simulink model "PLL_vs_Hilbert_Mdpi"  (R2024b)
settings: Solver=ode4  StartTime=0.0  StopTime=t(end)  FixedStep=dt  MaxStep=1/10  MinStep=1/10/100  RelTol=1e-3
values from neighbouring files (symbols this model uses):
  case_input = 4    [PLL_script_MDPI.m]
  dt = 1/Fs    (= 0.2)    [Excitation_Force_RM3.m]    (also in PLL_script_MDPI.m = t(2)-t(1); RM3_instf_init.m = round(t(2)-t(1),1); eta2Fex.m = 1/opt.Fs)
  H_s = 2    [PLL_script_MDPI.m]    (also in RM3_instf_init.m)
  median_window = round(2*delay_factor*window_size)    [PLL_script_MDPI.m]    (also in RM3_instf_init.m)
  median_window_seconds = round(0.05*window_size*dt)    [PLL_script_MDPI.m]
  wbar = 2*pi*fp    (= 0.698131700798)    [PLL_script_MDPI.m]    (also in RM3_instf_init.m)
  window_size = round(10*2*pi/wbar/dt)    [PLL_script_MDPI.m]    (also in RM3_instf_init.m)
undefined symbols (not defined in the file or in its folder): A_VCO, window_size_seconds
libraries: simulink x5, dspsigops x4, slpidlib x3, dspxfrm3 x3, dspfdesign x1, dspstat3 x1, eeSinusoidalMeasurementV2 x1
settings Model: Creator=inyongkim  LastModifiedBy=inyongkim
settings OptimizationCC: BlockReduction=off  DefaultParameterBehavior=Inlined  BufferReuse=off

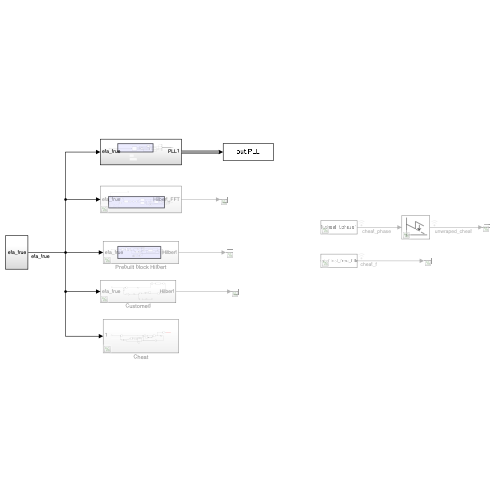
[thumbnail: Simulink's stored preview of the top-level diagram]
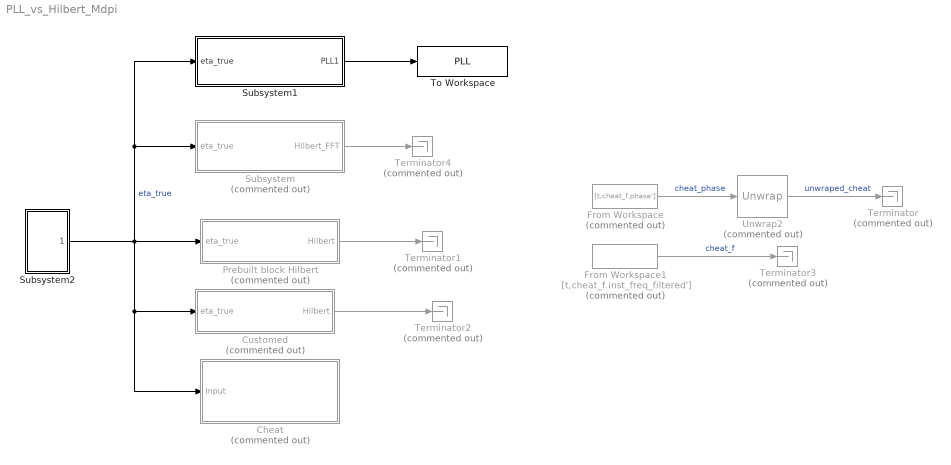
== system PLL_vs_Hilbert_Mdpi ==
  Cheat : Subsystem  Commented=on
  Customed : Subsystem  Commented=on
  From Workspace : FromWorkspace  Commented=on  VariableName=[t,cheat_f.phase']
  From Workspace1 : FromWorkspace  Commented=on  VariableName=[t,cheat_f.inst_freq_filtered']
  Prebuilt block Hilbert : Subsystem  Commented=on
  Subsystem : Subsystem  Commented=on
  Subsystem1 : Subsystem
  Subsystem2 : Subsystem
  Terminator{,1..4} (5 alike) : Terminator  Commented=on
  To Workspace : ToWorkspace  VariableName=PLL  SaveFormat=Timeseries  SampleTime=-1
  Unwrap2 : dspsigops/Unwrap  Commented=on  tol=pi  InputProcessing=Columns as channels (frame based)  running=off
  wires:
  Subsystem/1(Hilbert_FFT) -> Terminator4/1
  Prebuilt block Hilbert/1(Hilbert) -> Terminator1/1
  Subsystem1/1(PLL1) -> To Workspace/1
  Customed/1(Hilbert) -> Terminator2/1
  Subsystem2/1(eta_true) -> Cheat/1(Input), Customed/1(eta_true), Subsystem1/1(eta_true), Subsystem/1(eta_true), Prebuilt block Hilbert/1(eta_true)  "eta_true"
  From Workspace/1 -> Unwrap2/1  "cheat_phase"
  Unwrap2/1 -> Terminator/1  "unwraped_cheat"
  From Workspace1/1 -> Terminator3/1  "cheat_f"

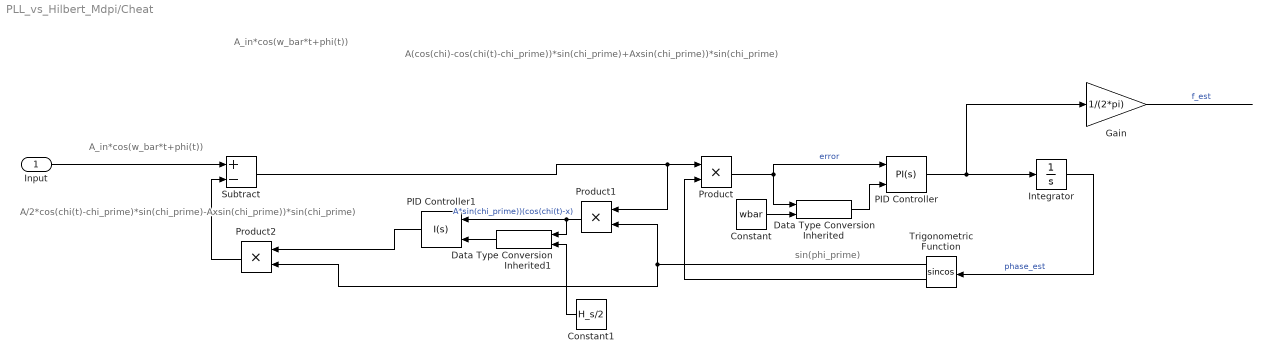
== system PLL_vs_Hilbert_Mdpi/Cheat ==
  note: A/2*cos(chi(t)-chi_prime)*sin(chi_prime)-Axsin(chi_prime))*sin(chi_prime)
  note: sin(phi_prime)
  note: A_in*cos(w_bar*t+phi(t))
  note: A_in*cos(w_bar*t+phi(t))
  note: A(cos(chi)-cos(chi(t)-chi_prime))*sin(chi_prime)+Axsin(chi_prime))*sin(chi_prime)
  Input : Inport
  Constant : Constant  Value=wbar
  Constant1 : Constant  Value=H_s/2
  Data Type Conversion Inherited : simulink/Signal Attributes/Data Type Conversion Inherited  ConvertRealWorld=Real World Value  DoSatur=off
  Data Type Conversion Inherited1 : simulink/Signal Attributes/Data Type Conversion Inherited  ConvertRealWorld=Real World Value  DoSatur=off
  Gain : Gain  Gain=1/(2*pi)
  Integrator : Integrator  LimitOutput=on  UpperSaturationLimit=2*pi  LowerSaturationLimit=0
  PID Controller : slpidlib/PID Controller  Controller=PI  Form=Parallel  TimeDomain=Continuous-time  UseExternalTs=off  SampleTime=-1  IntegratorMethod=Forward Euler  FilterMethod=Forward Euler  ControllerParametersSource=internal  P=1  I=1  UseKiTs=off  D=0  UseExternalDerivativeSource=off  N=100  UseFilter=on  TunerSelectOption=Transfer Function Based (PID Tuner App)  InitialConditionSource=external  InitialConditionForIntegrator=0  InitialConditionForFilter=0  DifferentiatorICPrevScaledInput=0  ExternalReset=none  TrackingMode=off  Kt=1  LimitOutput=on  SatLimitsSource=internal  UpperSaturationLimit=inf  LowerSaturationLimit=-inf  LinearizeAsGain=on  AntiWindupMode=clamping  Kb=1  LimitIntegrator=off  UpperIntegratorSaturationLimit=inf  LowerIntegratorSaturationLimit=-inf  POutMin=[]  POutMax=[]  IOutMin=[]  IOutMax=[]  DOutMin=[]  DOutMax=[]  NOutMin=[]  NOutMax=[]  SumOutMin=[]  SumOutMax=[]  SaturationOutMin=[]  SaturationOutMax=[]  PParamMin=[]  PParamMax=[]  IParamMin=[]  IParamMax=[]  DParamMin=[]  DParamMax=[]  NParamMin=[]  NParamMax=[]  KbParamMin=[]  KbParamMax=[]  KtParamMin=[]  KtParamMax=[]  KbOutMin=[]  KbOutMax=[]  KtOutMin=[]  KtOutMax=[]  IntegratorOutMin=[]  IntegratorOutMax=[]  FilterOutMin=[]  FilterOutMax=[]  SumI1OutMin=[]  SumI1OutMax=[]  SumI2OutMin=[]  SumI2OutMax=[]  SumI3OutMin=[]  SumI3OutMax=[]  SumI4OutMin=[]  SumI4OutMax=[]  SumDOutMin=[]  SumDOutMax=[]  DifferentiatorOutMin=[]  DifferentiatorOutMax=[]  FilterDiffOutCoefMin=[]  FilterDiffOutCoefMax=[]  ReciprocalOutMin=[]  ReciprocalOutMax=[]  SumDenOutMin=[]  SumDenOutMax=[]  SumNumOutMin=[]  SumNumOutMax=[]  DivideOutMin=[]  DivideOutMax=[]  UdiffTsProdOutMin=[]  UdiffTsProdOutMax=[]  NTsProdOutMin=[]  NTsProdOutMax=[]  UintegralTsProdOutMin=[]  UintegralTsProdOutMax=[]  UngainTsProdOutMin=[]  UngainTsProdOutMax=[]  ClampingZeroOutDataTypeStr=Inherit: Inherit via back propagation  ClampingZeroOutMin=[]  ClampingZeroOutMax=[]  FilterDenConstantOutDataTypeStr=Inherit: Inherit via back propagation  FilterDenConstantOutMin=[]  FilterDenConstantOutMax=[]  PCopyOutDataTypeStr=Inherit: Inherit via back propagation  PCopyOutMin=[]  PCopyOutMax=[]  NCopyOutDataTypeStr=Inherit: Inherit via back propagation  NCopyOutMin=[]  NCopyOutMax=[]  IntegratorContinuousStateAttributes=''  IntegratorStateMustResolveToSignalObject=off  IntegratorRTWStateStorageClass=Auto  FilterContinuousStateAttributes=''  FilterStateMustResolveToSignalObject=off  FilterRTWStateStorageClass=Auto  ParallelPVariant=InternalParameters  IdealPVariant=Disabled  IVariant=InternalParameters  DVariant=Disabled  IntegratorVariant=Continuous  SatVariant=Enabled  AWVariant=ContClampingParallel  PCopyVariant=Disabled  TRVariant=Disabled  FdbkBlocksVariant=Forward  IdealPFdbkVariant=Disabled  SatFdbkVariant=Disabled  DerivativeFilterVariant=Disabled  NVariant=Disabled  NCopyVariant=Disabled_SignalSpec  FilterICVariant=Disabled  IntegratorICVariant=ExternalICs  ExternalResetVariant=Disabled  TRSumVariant=Passthrough  SumFdbkVariant=Disabled  SumVariant=Sum_PI  TsampFilterVariant=InternalTs  TsampNgainVariant=Passthrough  TsampIntegralVariant=Disabled_SignalSpec  ExternalSaturationOutDataTypeStr=Inherit: Same as second input  DerivativeSourceVariant=Disabled  PreIntVariant=InternalPreInt
  PID Controller1 : slpidlib/PID Controller  Controller=I  Form=Parallel  TimeDomain=Continuous-time  UseExternalTs=off  SampleTime=-1  IntegratorMethod=Forward Euler  FilterMethod=Forward Euler  ControllerParametersSource=internal  P=1  I=1  UseKiTs=off  D=0  UseExternalDerivativeSource=off  N=100  UseFilter=on  TunerSelectOption=Transfer Function Based (PID Tuner App)  InitialConditionSource=external  InitialConditionForIntegrator=0  InitialConditionForFilter=0  DifferentiatorICPrevScaledInput=0  ExternalReset=none  TrackingMode=off  Kt=1  LimitOutput=on  SatLimitsSource=internal  UpperSaturationLimit=inf  LowerSaturationLimit=-inf  LinearizeAsGain=on  AntiWindupMode=clamping  Kb=1  LimitIntegrator=off  UpperIntegratorSaturationLimit=inf  LowerIntegratorSaturationLimit=-inf  POutMin=[]  POutMax=[]  IOutMin=[]  IOutMax=[]  DOutMin=[]  DOutMax=[]  NOutMin=[]  NOutMax=[]  SumOutMin=[]  SumOutMax=[]  SaturationOutMin=[]  SaturationOutMax=[]  PParamMin=[]  PParamMax=[]  IParamMin=[]  IParamMax=[]  DParamMin=[]  DParamMax=[]  NParamMin=[]  NParamMax=[]  KbParamMin=[]  KbParamMax=[]  KtParamMin=[]  KtParamMax=[]  KbOutMin=[]  KbOutMax=[]  KtOutMin=[]  KtOutMax=[]  IntegratorOutMin=[]  IntegratorOutMax=[]  FilterOutMin=[]  FilterOutMax=[]  SumI1OutMin=[]  SumI1OutMax=[]  SumI2OutMin=[]  SumI2OutMax=[]  SumI3OutMin=[]  SumI3OutMax=[]  SumI4OutMin=[]  SumI4OutMax=[]  SumDOutMin=[]  SumDOutMax=[]  DifferentiatorOutMin=[]  DifferentiatorOutMax=[]  FilterDiffOutCoefMin=[]  FilterDiffOutCoefMax=[]  ReciprocalOutMin=[]  ReciprocalOutMax=[]  SumDenOutMin=[]  SumDenOutMax=[]  SumNumOutMin=[]  SumNumOutMax=[]  DivideOutMin=[]  DivideOutMax=[]  UdiffTsProdOutMin=[]  UdiffTsProdOutMax=[]  NTsProdOutMin=[]  NTsProdOutMax=[]  UintegralTsProdOutMin=[]  UintegralTsProdOutMax=[]  UngainTsProdOutMin=[]  UngainTsProdOutMax=[]  ClampingZeroOutDataTypeStr=Inherit: Inherit via back propagation  ClampingZeroOutMin=[]  ClampingZeroOutMax=[]  FilterDenConstantOutDataTypeStr=Inherit: Inherit via back propagation  FilterDenConstantOutMin=[]  FilterDenConstantOutMax=[]  PCopyOutDataTypeStr=Inherit: Inherit via back propagation  PCopyOutMin=[]  PCopyOutMax=[]  NCopyOutDataTypeStr=Inherit: Inherit via back propagation  NCopyOutMin=[]  NCopyOutMax=[]  IntegratorContinuousStateAttributes=''  IntegratorStateMustResolveToSignalObject=off  IntegratorRTWStateStorageClass=Auto  FilterContinuousStateAttributes=''  FilterStateMustResolveToSignalObject=off  FilterRTWStateStorageClass=Auto  ParallelPVariant=Disabled  IdealPVariant=Disabled  IVariant=InternalParameters  DVariant=Disabled  IntegratorVariant=Continuous  SatVariant=Enabled  AWVariant=ContClampingParallel  PCopyVariant=Disabled  TRVariant=Disabled  FdbkBlocksVariant=Forward  IdealPFdbkVariant=Disabled  SatFdbkVariant=Disabled  DerivativeFilterVariant=Disabled  NVariant=Disabled  NCopyVariant=Disabled_SignalSpec  FilterICVariant=Disabled  IntegratorICVariant=ExternalICs  ExternalResetVariant=Disabled  TRSumVariant=Passthrough  SumFdbkVariant=Disabled  SumVariant=Passthrough_I  TsampFilterVariant=InternalTs  TsampNgainVariant=Passthrough  TsampIntegralVariant=Disabled_SignalSpec  ExternalSaturationOutDataTypeStr=Inherit: Same as second input  DerivativeSourceVariant=Disabled  PreIntVariant=InternalPreInt
  Product : Product
  Product1 : Product
  Product2 : Product
  Subtract : Sum  Inputs=+-
  Trigonometric Function : Trigonometry  Operator=sincos
  wires:
  PID Controller/1 -> Gain/1, Integrator/1
  Trigonometric Function/2 -> Product/2
  Input/1 -> Subtract/1
  Subtract/1 -> Product1/1, Product/1
  Product1/1 -> Data Type Conversion Inherited1/1, PID Controller1/1  "A*sin(chi_prime))(cos(chi(t)-x)"
  Trigonometric Function/1 -> Product1/2, Product2/2
  PID Controller1/1 -> Product2/1
  Product2/1 -> Subtract/2
  Product/1 -> Data Type Conversion Inherited/1, PID Controller/1  "error"
  Integrator/1 -> Trigonometric Function/1  "phase_est"
  Gain/1 -> ?  "f_est"
  Constant/1 -> Data Type Conversion Inherited/2
  Data Type Conversion Inherited/1 -> PID Controller/2
  Data Type Conversion Inherited1/1 -> PID Controller1/2
  Constant1/1 -> Data Type Conversion Inherited1/2

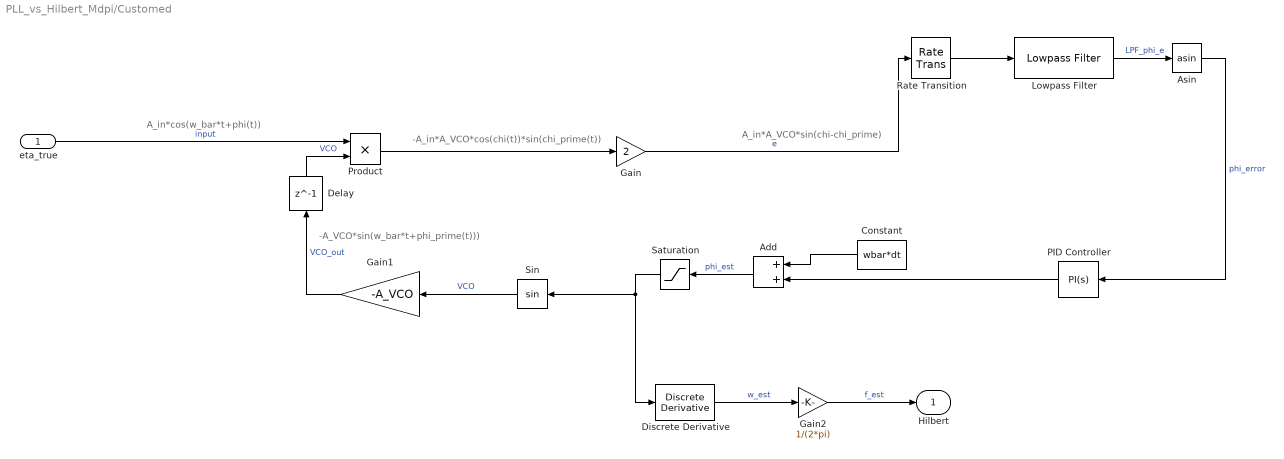
== system PLL_vs_Hilbert_Mdpi/Customed ==
  note: A_in*cos(w_bar*t+phi(t))
  note: -A_VCO*sin(w_bar*t+phi_prime(t)))
  note: -A_in*A_VCO*cos(chi(t))*sin(chi_prime(t))
  note: A_in*A_VCO*sin(chi-chi_prime)
  eta_true : Inport
  Add : Sum
  Asin : Trigonometry  Operator=asin
  Constant : Constant  Value=wbar*dt
  Delay : Delay  DelayLength=1  InitialCondition=-0.5
  Discrete Derivative : simulink/Discrete/Discrete Derivative  gainval=1.0  ICPrevScaledInput=0.0  OutMin=[]  OutMax=[]  OutDataType=fixdt(1, 16)  OutScaling=2^-10  DoSatur=off
  Gain : Gain  Gain=2
  Gain1 : Gain  Gain=-A_VCO
  Gain2 : Gain  Gain=1/(2*pi)
  Lowpass Filter : dspfdesign/Lowpass Filter  FilterType=FIR  DesignForMinimumOrder=on  FilterOrder=50  PassbandFrequency=wbar/2/pi  StopbandFrequency=wbar/pi  PassbandRipple=0.5  StopbandAttenuation=40  SampleRate=100  SimulateUsing=Interpreted execution  roundingMode=Floor  coeffsDataTypeStr=fixdt(1,16)
  PID Controller : slpidlib/PID Controller  Controller=PI  Form=Parallel  TimeDomain=Continuous-time  UseExternalTs=off  SampleTime=-1  IntegratorMethod=Forward Euler  FilterMethod=Forward Euler  ControllerParametersSource=internal  P=0  I=1  UseKiTs=off  D=0  UseExternalDerivativeSource=off  N=100  UseFilter=on  TunerSelectOption=Transfer Function Based (PID Tuner App)  InitialConditionSource=internal  InitialConditionForIntegrator=0  InitialConditionForFilter=0  DifferentiatorICPrevScaledInput=0  ExternalReset=none  TrackingMode=off  Kt=1  LimitOutput=on  SatLimitsSource=internal  UpperSaturationLimit=pi  LowerSaturationLimit=-pi  LinearizeAsGain=on  AntiWindupMode=back-calculation  Kb=1  LimitIntegrator=off  UpperIntegratorSaturationLimit=inf  LowerIntegratorSaturationLimit=-inf  POutMin=[]  POutMax=[]  IOutMin=[]  IOutMax=[]  DOutMin=[]  DOutMax=[]  NOutMin=[]  NOutMax=[]  SumOutMin=[]  SumOutMax=[]  SaturationOutMin=[]  SaturationOutMax=[]  PParamMin=[]  PParamMax=[]  IParamMin=[]  IParamMax=[]  DParamMin=[]  DParamMax=[]  NParamMin=[]  NParamMax=[]  KbParamMin=[]  KbParamMax=[]  KtParamMin=[]  KtParamMax=[]  KbOutMin=[]  KbOutMax=[]  KtOutMin=[]  KtOutMax=[]  IntegratorOutMin=[]  IntegratorOutMax=[]  FilterOutMin=[]  FilterOutMax=[]  SumI1OutMin=[]  SumI1OutMax=[]  SumI2OutMin=[]  SumI2OutMax=[]  SumI3OutMin=[]  SumI3OutMax=[]  SumI4OutMin=[]  SumI4OutMax=[]  SumDOutMin=[]  SumDOutMax=[]  DifferentiatorOutMin=[]  DifferentiatorOutMax=[]  FilterDiffOutCoefMin=[]  FilterDiffOutCoefMax=[]  ReciprocalOutMin=[]  ReciprocalOutMax=[]  SumDenOutMin=[]  SumDenOutMax=[]  SumNumOutMin=[]  SumNumOutMax=[]  DivideOutMin=[]  DivideOutMax=[]  UdiffTsProdOutMin=[]  UdiffTsProdOutMax=[]  NTsProdOutMin=[]  NTsProdOutMax=[]  UintegralTsProdOutMin=[]  UintegralTsProdOutMax=[]  UngainTsProdOutMin=[]  UngainTsProdOutMax=[]  ClampingZeroOutDataTypeStr=Inherit: Inherit via back propagation  ClampingZeroOutMin=[]  ClampingZeroOutMax=[]  FilterDenConstantOutDataTypeStr=Inherit: Inherit via back propagation  FilterDenConstantOutMin=[]  FilterDenConstantOutMax=[]  PCopyOutDataTypeStr=Inherit: Inherit via back propagation  PCopyOutMin=[]  PCopyOutMax=[]  NCopyOutDataTypeStr=Inherit: Inherit via back propagation  NCopyOutMin=[]  NCopyOutMax=[]  IntegratorContinuousStateAttributes=''  IntegratorStateMustResolveToSignalObject=off  IntegratorRTWStateStorageClass=Auto  FilterContinuousStateAttributes=''  FilterStateMustResolveToSignalObject=off  FilterRTWStateStorageClass=Auto  ParallelPVariant=InternalParameters  IdealPVariant=Disabled  IVariant=InternalParameters  DVariant=Disabled  IntegratorVariant=Continuous  SatVariant=Enabled  AWVariant=BackCalculation  PCopyVariant=Disabled  TRVariant=Disabled  FdbkBlocksVariant=Forward  IdealPFdbkVariant=Disabled  SatFdbkVariant=Disabled  DerivativeFilterVariant=Disabled  NVariant=Disabled  NCopyVariant=Disabled_SignalSpec  FilterICVariant=Disabled  IntegratorICVariant=InternalICs  ExternalResetVariant=Disabled  TRSumVariant=Passthrough  SumFdbkVariant=Disabled  SumVariant=Sum_PI  TsampFilterVariant=InternalTs  TsampNgainVariant=Passthrough  TsampIntegralVariant=Disabled_SignalSpec  ExternalSaturationOutDataTypeStr=Inherit: Same as second input  DerivativeSourceVariant=Disabled  PreIntVariant=InternalPreInt
  Product : Product
  Rate Transition : RateTransition  OutPortSampleTimeOpt=Inherit
  Saturation : Saturate  UpperLimit=pi  LowerLimit=-pi
  Sin : Trigonometry
  Hilbert : Outport
  wires:
  Product/1 -> Gain/1
  Asin/1 -> PID Controller/1  "phi_error"
  eta_true/1 -> Product/1  "input"
  Gain1/1 -> Delay/1  "VCO_out"
  Sin/1 -> Gain1/1  "VCO"
  Gain/1 -> Rate Transition/1  "e"
  Discrete Derivative/1 -> Gain2/1  "w_est"
  Gain2/1 -> Hilbert/1  "f_est"
  Lowpass Filter/1 -> Asin/1  "LPF_phi_e"
  Rate Transition/1 -> Lowpass Filter/1
  Constant/1 -> Add/1
  Add/1 -> Saturation/1  "phi_est"
  Delay/1 -> Product/2  "VCO"
  Saturation/1 -> Discrete Derivative/1, Sin/1
  PID Controller/1 -> Add/2

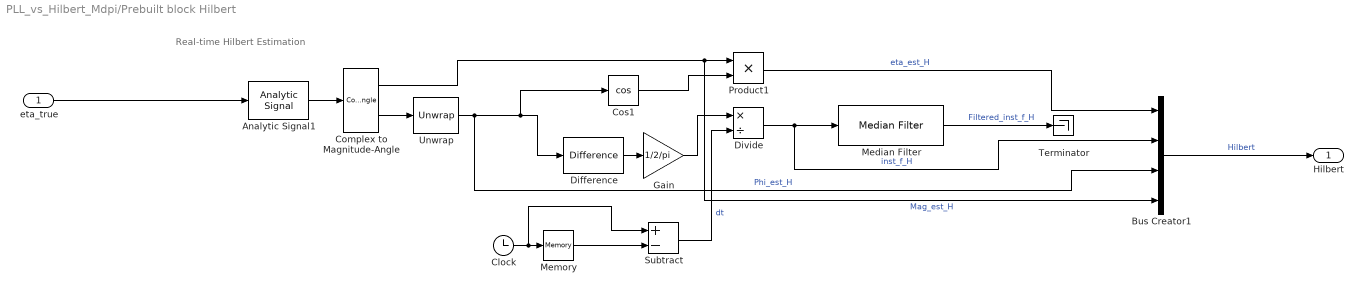
== system PLL_vs_Hilbert_Mdpi/Prebuilt block Hilbert ==
  note: Real-time Hilbert Estimation
  eta_true : Inport
  Analytic Signal1 : dspxfrm3/Analytic Signal  N=30  InputProcessing=Columns as channels (frame based)
  Bus Creator1 : BusCreator  Inputs=4
  Clock : Clock
  Complex to Magnitude-Angle : ComplexToMagnitudeAngle
  Cos1 : Trigonometry  Operator=cos
  Difference : simulink/Discrete/Difference  ICPrevInput=0.0  OutMin=[]  OutMax=[]  OutDataType=fixdt(1, 16)  OutScaling=2^-10  DoSatur=off
  Divide : Product  Inputs=*/
  Gain : Gain  Gain=1/2/pi
  Median Filter : dspstat3/Median Filter  WindowLength=round(median_window_seconds/dt)  SimulateUsing=Interpreted execution
      settings: LibrarySourceBlock=|
      | dspfdesign/Median
      | Filter
  Memory : Memory
  Product1 : Product
  Subtract : Sum  Inputs=+-
  Terminator : Terminator
  Unwrap : dspsigops/Unwrap  tol=pi  InputProcessing=Columns as channels (frame based)  running=off
  Hilbert : Outport
  wires:
  eta_true/1 -> Analytic Signal1/1
  Median Filter/1 -> Terminator/1  "Filtered_inst_f_H"
  Cos1/1 -> Product1/2
  Memory/1 -> Subtract/2
  Divide/1 -> Bus Creator1/2, Median Filter/1  "inst_f_H"
  Subtract/1 -> Divide/2  "dt"
  Analytic Signal1/1 -> Complex to Magnitude-Angle/1
  Product1/1 -> Bus Creator1/1  "eta_est_H"
  Gain/1 -> Divide/1
  Clock/1 -> Subtract/1, Memory/1
  Bus Creator1/1 -> Hilbert/1  "Hilbert"
  Complex to Magnitude-Angle/2 -> Unwrap/1
  Unwrap/1 -> Bus Creator1/3, Cos1/1, Difference/1  "Phi_est_H"
  Difference/1 -> Gain/1
  Complex to Magnitude-Angle/1 -> Bus Creator1/4, Product1/1  "Mag_est_H"

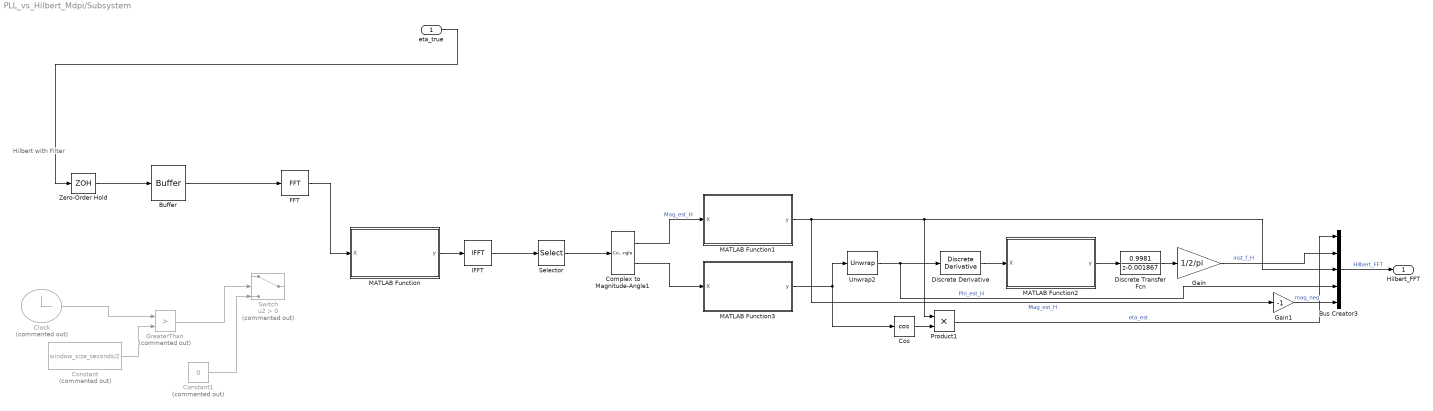
== system PLL_vs_Hilbert_Mdpi/Subsystem ==
  note: Hilbert with Filter
  eta_true : Inport
  Buffer : Buffer  N=window_size  V=window_size-1  OutputFrames=off
  Bus Creator3 : BusCreator  Inputs=5
  Clock : Clock  Commented=on
      settings: Decimation=window_size_seconds
  Complex to Magnitude-Angle1 : ComplexToMagnitudeAngle
  Constant : Constant  Commented=on  Value=window_size_seconds/2
  Constant1 : Constant  Commented=on  Value=0
  Cos : Trigonometry  Operator=cos
  Discrete Transfer Fcn : DiscreteTransferFcn  Numerator=[0.9981]  Denominator=[1 -0.001867]
  Discrete Derivative : simulink/Quick Insert/Discrete/Discrete Derivative  gainval=1.0  ICPrevScaledInput=0.0  OutMin=[]  OutMax=[]  OutDataType=fixdt(1, 16)  OutScaling=2^-10  DoSatur=off
  FFT : dspxfrm3/FFT  FFTImplementation=Auto  CompMethod=Table lookup  TableOpt=NEW  TableOptActive=Speed  BitRevOrder=off  Normalize=off  InheritFFTLength=on  FFTLength=64  WrapInput=on  roundingMode=Ceiling  overflowMode=off  firstCoeffDataTypeStr=Inherit: Same word length as input  firstCoeffLastDataTypeStr=Inherit: Same word length as input  outputMin=[]  outputMax=[]
  Gain : Gain  Gain=1/2/pi
  Gain1 : Gain  Gain=-1
  GreaterThan : RelationalOperator  Commented=on  Operator=>  OutDataTypeStr=boolean  RndMeth=Simplest  InputSameDT=off
  IFFT : dspxfrm3/IFFT  FFTImplementation=Auto  CompMethod=Table lookup  TableOpt=NEW  TableOptActive=Speed  BitRevOrder=off  cs_in=off  Normalize=on  InheritFFTLength=on  FFTLength=100  WrapInput=on  mode=Real  outSamplingMode=Sample based  roundingMode=Ceiling  overflowMode=off  firstCoeffDataTypeStr=Inherit: Same word length as input  firstCoeffLastDataTypeStr=Inherit: Same word length as input  outputMin=[]  outputMax=[]
  MATLAB Function : MATLAB Function  TreatAsAtomicUnit=on
  MATLAB Function1 : MATLAB Function  TreatAsAtomicUnit=on
  MATLAB Function2 : MATLAB Function  TreatAsAtomicUnit=on
  MATLAB Function3 : MATLAB Function  TreatAsAtomicUnit=on
  Product1 : Product
  Selector : Selector  InputPortWidth=window_size  IndexOptions=Index vector (dialog)  Indices=[window_size-median_window:window_size]  OutputSizes=1
  Switch : Switch  Commented=on  Criteria=u2 > Threshold  SaturateOnIntegerOverflow=off  InputSameDT=off
  Unwrap2 : dspsigops/Unwrap  tol=pi  InputProcessing=Columns as channels (frame based)  running=off
  Zero-Order Hold : ZeroOrderHold  SampleTime=dt
  Hilbert_FFT : Outport
  wires:
  Bus Creator3/1 -> Hilbert_FFT/1  "Hilbert_FFT"
  eta_true/1 -> Zero-Order Hold/1
  Gain1/1 -> Bus Creator3/5  "mag_neg"
  MATLAB Function2/1(y) -> Discrete Transfer Fcn/1
  Selector/1 -> Complex to Magnitude-Angle1/1
  MATLAB Function/1(y) -> IFFT/1
  Constant1/1 -> Switch/3
  Unwrap2/1 -> Bus Creator3/4, Discrete Derivative/1  "Phi_est_H"
  GreaterThan/1 -> Switch/2
  Gain/1 -> Bus Creator3/2  "inst_f_H"
  Discrete Transfer Fcn/1 -> Gain/1
  Constant/1 -> GreaterThan/2
  Complex to Magnitude-Angle1/1 -> MATLAB Function1/1(X)  "Mag_est_H"
  Product1/1 -> Bus Creator3/1  "eta_est"
  Clock/1 -> GreaterThan/1
  IFFT/1 -> Selector/1
  MATLAB Function3/1(y) -> Unwrap2/1, Cos/1
  Discrete Derivative/1 -> MATLAB Function2/1(X)
  Complex to Magnitude-Angle1/2 -> MATLAB Function3/1(X)
  Buffer/1 -> FFT/1
  Zero-Order Hold/1 -> Buffer/1
  MATLAB Function1/1(y) -> Bus Creator3/3, Product1/1, Gain1/1  "Mag_est_H"
  FFT/1 -> MATLAB Function/1(X)
  Cos/1 -> Product1/2

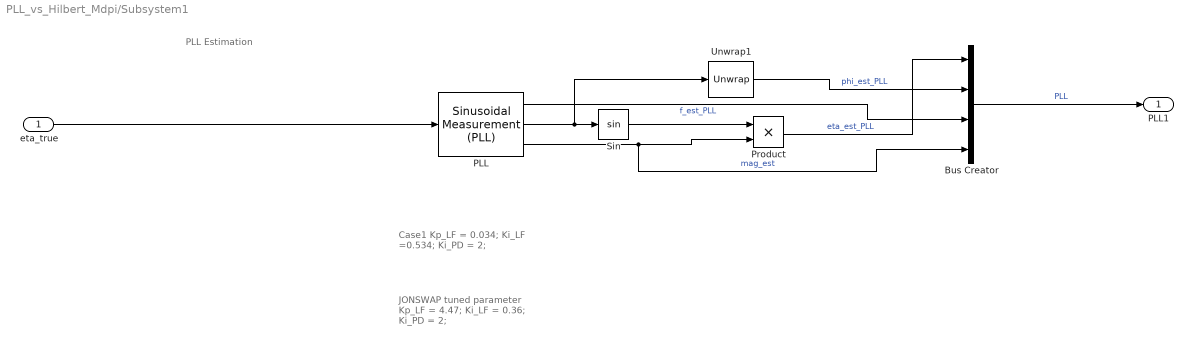
== system PLL_vs_Hilbert_Mdpi/Subsystem1 ==
  note: JONSWAP tuned parameter
      | Kp_LF = 4.47;
      | Ki_LF = 0.36;
      | Ki_PD = 2;
  note: PLL Estimation
  note: Case1
      | Kp_LF = 0.034;
      | Ki_LF =0.534;
      | Ki_PD = 2;
  eta_true : Inport
  Bus Creator : BusCreator  Inputs=4
  PLL : eeSinusoidalMeasurementV2/Sinusoidal Measurement (PLL)  Ki_PD=2  Kp_LF=Kp_LF  Ki_LF=Ki_LF  F0=wbar/2/pi  Theta0=0  Mag0=1  Ts=-1
      settings: LibrarySourceBlock=|
      | ee_sl_lib/Measurements/Sinusoidal Measurement
      | (PLL)
  Product : Product
  Sin : Trigonometry
  Unwrap1 : dspsigops/Unwrap  tol=pi  running=off
  PLL1 : Outport
  wires:
  Unwrap1/1 -> Bus Creator/2  "phi_est_PLL"
  Product/1 -> Bus Creator/1  "eta_est_PLL"
  eta_true/1 -> PLL/1
  PLL/2 -> Unwrap1/1, Sin/1
  Sin/1 -> Product/1
  PLL/1 -> Bus Creator/3  "f_est_PLL"
  Bus Creator/1 -> PLL1/1  "PLL"
  PLL/3 -> Bus Creator/4, Product/2  "mag_est"

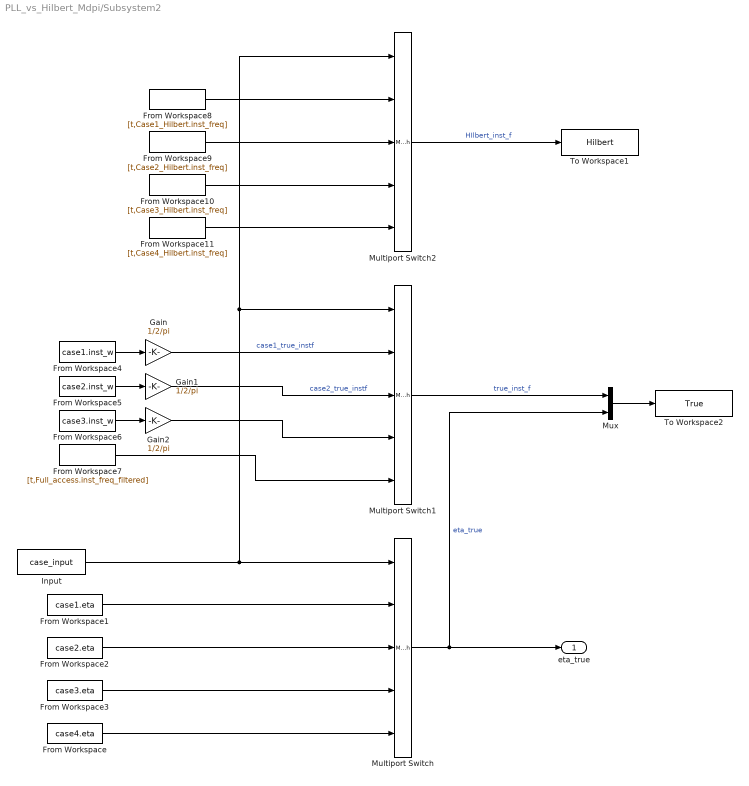
== system PLL_vs_Hilbert_Mdpi/Subsystem2 ==
  From Workspace : FromWorkspace  VariableName=case4.eta
  From Workspace1 : FromWorkspace  VariableName=case1.eta
  From Workspace10 : FromWorkspace  VariableName=[t,Case3_Hilbert.inst_freq]
  From Workspace11 : FromWorkspace  VariableName=[t,Case4_Hilbert.inst_freq]
  From Workspace2 : FromWorkspace  VariableName=case2.eta
  From Workspace3 : FromWorkspace  VariableName=case3.eta
  From Workspace4 : FromWorkspace  VariableName=case1.inst_w
  From Workspace5 : FromWorkspace  VariableName=case2.inst_w
  From Workspace6 : FromWorkspace  VariableName=case3.inst_w
  From Workspace7 : FromWorkspace  VariableName=[t,Full_access.inst_freq_filtered]
  From Workspace8 : FromWorkspace  VariableName=[t,Case1_Hilbert.inst_freq]
  From Workspace9 : FromWorkspace  VariableName=[t,Case2_Hilbert.inst_freq]
  Gain : Gain  Gain=1/2/pi
  Gain1 : Gain  Gain=1/2/pi
  Gain2 : Gain  Gain=1/2/pi
  Input : Constant  Value=case_input
  Multiport Switch : MultiPortSwitch  Inputs=4  SaturateOnIntegerOverflow=off  InputSameDT=off
  Multiport Switch1 : MultiPortSwitch  Inputs=4  SaturateOnIntegerOverflow=off  InputSameDT=off
  Multiport Switch2 : MultiPortSwitch  Inputs=4  SaturateOnIntegerOverflow=off  InputSameDT=off
  Mux : Mux  Inputs=2
  To Workspace1 : ToWorkspace  VariableName=Hilbert  SaveFormat=Timeseries  SampleTime=-1
  To Workspace2 : ToWorkspace  VariableName=True  SaveFormat=Timeseries  SampleTime=-1
  eta_true : Outport
  wires:
  Multiport Switch/1 -> Mux/2, eta_true/1  "eta_true"
  From Workspace/1 -> Multiport Switch/5
  From Workspace3/1 -> Multiport Switch/4
  Input/1 -> Multiport Switch1/1, Multiport Switch2/1, Multiport Switch/1
  From Workspace2/1 -> Multiport Switch/3
  From Workspace1/1 -> Multiport Switch/2
  From Workspace4/1 -> Gain/1
  From Workspace5/1 -> Gain1/1
  From Workspace6/1 -> Gain2/1
  Gain/1 -> Multiport Switch1/2  "case1_true_instf"
  Gain1/1 -> Multiport Switch1/3  "case2_true_instf"
  Gain2/1 -> Multiport Switch1/4
  From Workspace7/1 -> Multiport Switch1/5
  From Workspace11/1 -> Multiport Switch2/5
  From Workspace10/1 -> Multiport Switch2/4
  From Workspace9/1 -> Multiport Switch2/3
  From Workspace8/1 -> Multiport Switch2/2
  Multiport Switch2/1 -> To Workspace1/1  "HIlbert_inst_f"
  Multiport Switch1/1 -> Mux/1  "true_inst_f"
  Mux/1 -> To Workspace2/1

== matlab function PLL_vs_Hilbert_Mdpi/Subsystem/MATLAB Function ==
  data: X input; y output
function y = hilbert_transform(X)
    N = length(X);
    H = zeros(size(X)); % Hilbert transform filter
    H(1) = 1;           % DC component remains the same
    H(2:N/2) = 2;       % Positive frequencies are scaled by 2
    H(N/2+1:end) = 0;   % Negative frequencies are set to zero
    y = H .* X;         % Apply the filter
end

== matlab function PLL_vs_Hilbert_Mdpi/Subsystem/MATLAB Function2 ==
  data: X input; y output
function y = median_filter(X)
    % Declare persistent variables to hold previous values
    persistent xm1 xm2
    
    % Initialize the persistent variables on first run
    if isempty(xm1)
        xm1 = X; % Initialize with the first input
    end
    if isempty(xm2)
        xm2 = X; % Initialize with the first input
    end
    
    % Apply the 3-point median filter
    y = median([X, xm1, xm2]);
    
    % Update the persistent variables
    xm2 = xm1;  % Shift older value to xm2
    xm1 = X;    % Update xm1 with the current input
end

== matlab function PLL_vs_Hilbert_Mdpi/Subsystem/MATLAB Function3 ==
  data: X input; y output
function y = median(X)
    y = median(X);         % Apply the filter
end

== matlab function PLL_vs_Hilbert_Mdpi/Subsystem/MATLAB Function1 ==
  data: X input; y output
function y = median(X)
    y = median(X);         % Apply the filter
end
